simulink model "Car_FLC_Simulink"  (R2019a)
settings: Solver=VariableStepAuto  StartTime=0.0  StopTime=10.0  RelTol=1e-3
libraries: fuzblock x1, simulink x1
settings Model: Creator=Konstantinos  LastModifiedBy=Konstantinos

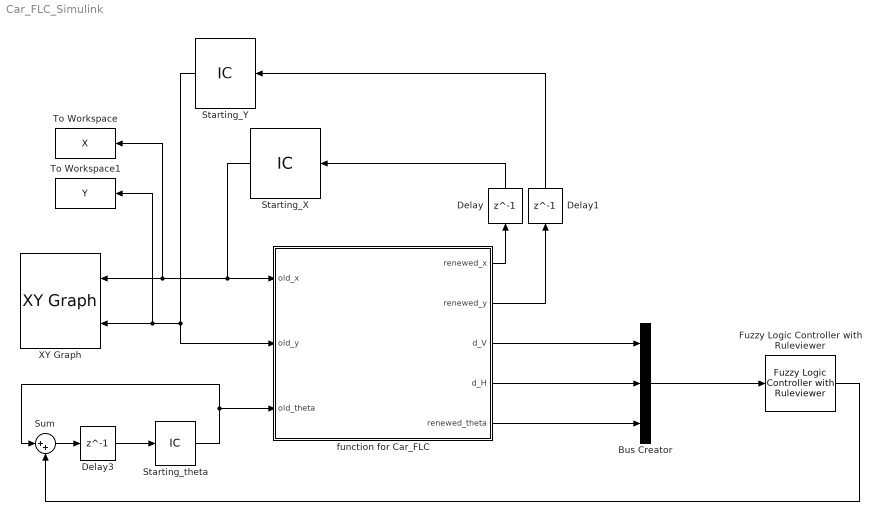
== system Car_FLC_Simulink ==
  Bus Creator : BusCreator  Inputs=3
  Delay : Delay  DelayLength=1  InitialCondition=0
  Delay1 : Delay  DelayLength=1  InitialCondition=0
  Delay3 : Delay  DelayLength=1  InitialCondition=0
  Fuzzy Logic Controller with Ruleviewer : fuzblock/Fuzzy Logic  Controller  with Ruleviewer  fismatrix=Car_FLC  Ts=0.01
  Starting_X : InitialCondition  Value=3.8
  Starting_Y : InitialCondition  Value=0.5
  Starting_theta : InitialCondition  Value=-45
  Sum : Sum  Inputs=|++
  To Workspace : ToWorkspace  VariableName=X  SampleTime=-1
  To Workspace1 : ToWorkspace  VariableName=Y  SampleTime=-1
  XY Graph : simulink/Sinks/XY Graph  xmin=0  xmax=10  ymin=0  ymax=4  st=-1
  function for Car_FLC : MATLAB Function  TreatAsAtomicUnit=on
  wires:
  Delay3/1 -> Starting_theta/1
  Sum/1 -> Delay3/1
  Starting_theta/1 -> Sum/1, function for Car_FLC/3(old_theta)
  Fuzzy Logic Controller with Ruleviewer/1 -> Sum/2
  Delay/1 -> Starting_X/1
  Bus Creator/1 -> Fuzzy Logic Controller with Ruleviewer/1
  Delay1/1 -> Starting_Y/1
  Starting_Y/1 -> function for Car_FLC/2(old_y), To Workspace1/1, XY Graph/2
  function for Car_FLC/5(renewed_theta) -> Bus Creator/3
  function for Car_FLC/1(renewed_x) -> Delay/1
  function for Car_FLC/4(d_H) -> Bus Creator/2
  function for Car_FLC/3(d_V) -> Bus Creator/1
  function for Car_FLC/2(renewed_y) -> Delay1/1
  Starting_X/1 -> XY Graph/1, To Workspace/1, function for Car_FLC/1(old_x)

== matlab function Car_FLC_Simulink/function for Car_FLC ==
  data: old_x input; renewed_x output; old_y input; old_theta input; renewed_y output; d_V output; d_H output; renewed_theta output
function [renewed_x, renewed_y, d_V, d_H, renewed_theta] = car_control(old_x, old_y, old_theta)
    my_theta = old_theta;
    renewed_theta = my_theta;
    
    % initial d_V and d_H in every round
    d_V = 0;
    d_H = 0;
    
    % krataw to theta apo -180 ews 180
    if ( my_theta < -180 )
        renewed_theta = my_theta + 360;
    end

    if( my_theta > 180 )
        renewed_theta = my_theta - 360;
    end


    % u
    u = 0.05;
    
    % vriskw ta nea x kai y
    this_x = u*cosd(my_theta);
    this_y = u*sin(my_theta);
    
    renewed_x = old_x + this_x;
    renewed_y = old_y + this_y;

    % ipologizw twra ta d_V kai ta d_H
    
    if (renewed_x < 5)
        d_V = renewed_y;
    elseif (renewed_x < 6)
        d_V = renewed_y - 1;
    elseif (renewed_x < 7)
        d_V = renewed_y - 2;
    elseif (renewed_x >= 7)
        d_V = renewed_y - 3;
    end
    
    if (renewed_y < 1)
        d_H = 5 - renewed_x;
    elseif (renewed_y < 2)
        d_H = 6 - renewed_x;
    elseif (renewed_y < 3)
        d_H = 7 - renewed_x;
    elseif (renewed_y >= 3)
        d_H = 1 ; % apeiri apostasi ousiastika
    end
    
    % Kanonikopoiw ta d_V kai d_H gia na ta valw mesa ston FLC
    
    if (d_V < 0)
        d_V = 0;
    elseif (d_V > 1)
        d_V = 1;
    end
    
     if (d_H < 0)
        d_H = 0;
    elseif (d_H > 1)
        d_H = 1;
     end
    
     
     
end
